simulink model "generator_voltage_control_delay"  (R2022b)
settings: Solver=VariableStepAuto  StartTime=0.0  StopTime=150.0  RelTol=1e-3
settings Model: Creator=Fabian  LastModifiedBy=Fabian

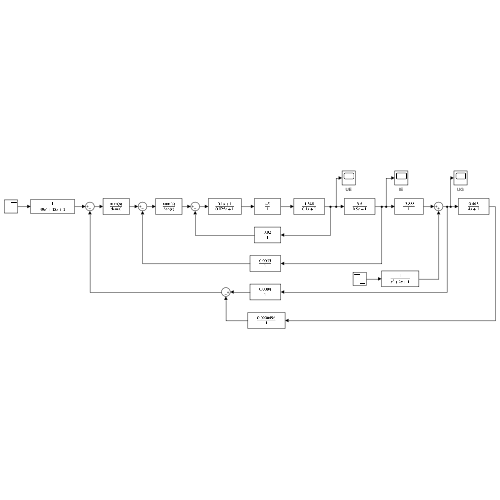
[thumbnail: Simulink's stored preview of the top-level diagram]
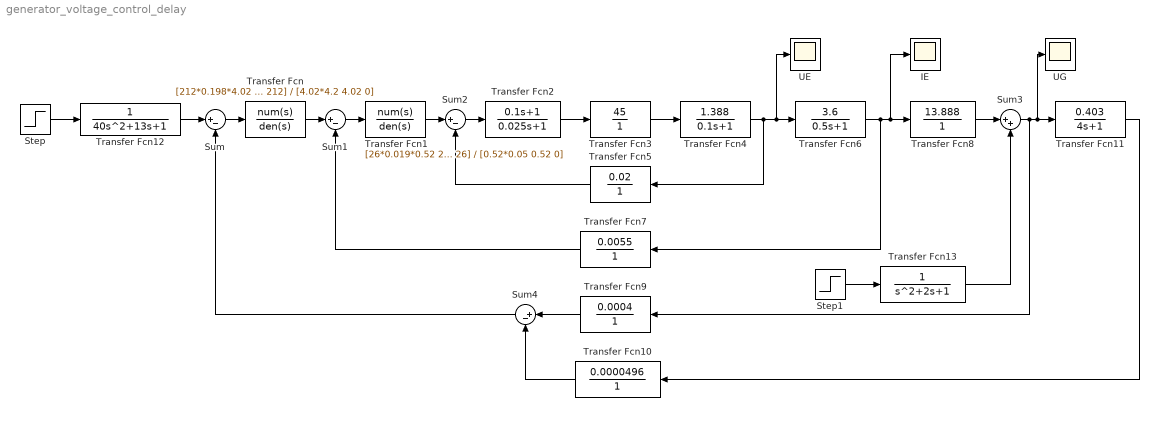
== system generator_voltage_control_delay ==
  IE : Scope
  Step : Step  Time=0  After=10  SampleTime=0
  Step1 : Step  Time=80  After=-1000  SampleTime=0
  Sum{,1..2,4} (4 alike) : Sum  Inputs=|+-
  Sum3 : Sum  Inputs=|++
  Transfer Fcn : TransferFcn  Numerator=[212*0.198*4.02 212*4.02 212]  Denominator=[4.02*4.2 4.02 0]
  Transfer Fcn1 : TransferFcn  Numerator=[26*0.019*0.52 26*0.52 26]  Denominator=[0.52*0.05 0.52 0]
  Transfer Fcn10 : TransferFcn  Numerator=[0.0000496]  Denominator=[1]
  Transfer Fcn11 : TransferFcn  Numerator=[0.403]  Denominator=[4 1]
  Transfer Fcn12 : TransferFcn  Denominator=[40 13 1]
  Transfer Fcn13 : TransferFcn
  Transfer Fcn2 : TransferFcn  Numerator=[0.1 1]  Denominator=[0.025 1]
  Transfer Fcn3 : TransferFcn  Numerator=[45]  Denominator=[1]
  Transfer Fcn4 : TransferFcn  Numerator=[1.388]  Denominator=[0.1 1]
  Transfer Fcn5 : TransferFcn  Numerator=[0.02]  Denominator=[1]
  Transfer Fcn6 : TransferFcn  Numerator=[3.6]  Denominator=[0.5 1]
  Transfer Fcn7 : TransferFcn  Numerator=[0.0055]  Denominator=[1]
  Transfer Fcn8 : TransferFcn  Numerator=[13.888]  Denominator=[1]
  Transfer Fcn9 : TransferFcn  Numerator=[0.0004]  Denominator=[1]
  UE : Scope
  UG : Scope
  wires:
  Transfer Fcn6/1 -> IE/1, Transfer Fcn8/1, Transfer Fcn7/1
  Transfer Fcn2/1 -> Transfer Fcn3/1
  Transfer Fcn7/1 -> Sum1/2
  Sum3/1 -> UG/1, Transfer Fcn11/1, Transfer Fcn9/1
  Transfer Fcn11/1 -> Transfer Fcn10/1
  Transfer Fcn8/1 -> Sum3/1
  Transfer Fcn9/1 -> Sum4/1
  Sum4/1 -> Sum/2
  Transfer Fcn/1 -> Sum1/1
  Transfer Fcn5/1 -> Sum2/2
  Sum/1 -> Transfer Fcn/1
  Transfer Fcn4/1 -> Transfer Fcn6/1, UE/1, Transfer Fcn5/1
  Transfer Fcn10/1 -> Sum4/2
  Sum1/1 -> Transfer Fcn1/1
  Transfer Fcn3/1 -> Transfer Fcn4/1
  Sum2/1 -> Transfer Fcn2/1
  Transfer Fcn1/1 -> Sum2/1
  Transfer Fcn12/1 -> Sum/1
  Step/1 -> Transfer Fcn12/1
  Step1/1 -> Transfer Fcn13/1
  Transfer Fcn13/1 -> Sum3/2
